simulink model "qiita3"  (R2019a)
settings: Solver=FixedStepDiscrete  StartTime=0.0  StopTime=Inf  FixedStep=0.001  RelTol=1e-3  EnableMultiTasking=on
libraries: robotlib x12, simulink x5
settings Model: Creator=tatsuyai  LastModifiedBy=tatsuyai
settings SolverCC: PositivePriorityOrder=on
settings OptimizationCC: EnhancedBackFolding=on  PassReuseOutputArgsAs=Individual arguments  ZeroExternalMemoryAtStartup=off  ZeroInternalMemoryAtStartup=off  MaxStackSize=64  OptimizeBlockOrder=speed  DifferentSizesBufferReuse=on  OptimizationCustomize=off
settings DebuggingCC: ParameterTunabilityLossMsg=error
settings HardwareCC: ProdBitPerLong=64  ProdBitPerPointer=32  ProdBitPerSizeT=32  ProdBitPerPtrDiffT=32  ProdLargestAtomicInteger=Long  ProdLargestAtomicFloat=Double  ProdWordSize=32  ProdHWDeviceType=ARM Compatible->ARM Cortex  TargetBitPerLong=64  UseEmbeddedCoderFeatures=off  UseSimulinkCoderFeatures=off
settings RTWCC: SystemTargetFile=ert.tlc  HardwareBoard=Raspberry Pi - Robot Operating System (ROS)  TLCOptions="-aInlineSetEventsForThisBaseRateFcn=TLC_FALSE -aSuppressMultiTaskScheduler=TLC_FALSE  -aRateBasedStepFcn=0"  TemplateMakefile=ert_default_tmf  GenerateReport=on  Toolchain=Catkin  BuildConfiguration=Faster Runs  IncludeHyperlinkInReport=on  LaunchReport=on  TargetLang=C++  GenerateTraceInfo=on  GenerateTraceReport=on  GenerateTraceReportSl=on  GenerateTraceReportSf=on  GenerateTraceReportEml=on
settings CodeAppCC: ForceParamTrailComments=on  IgnoreCustomStorageClasses=off  OperatorAnnotations=on  SimulinkDataObjDesc=on  SFDataObjDesc=on  InsertBlockDesc=on
settings ERTTargetCC: SupportNonInlinedSFcns=on  SupportVariableSizeSignals=on

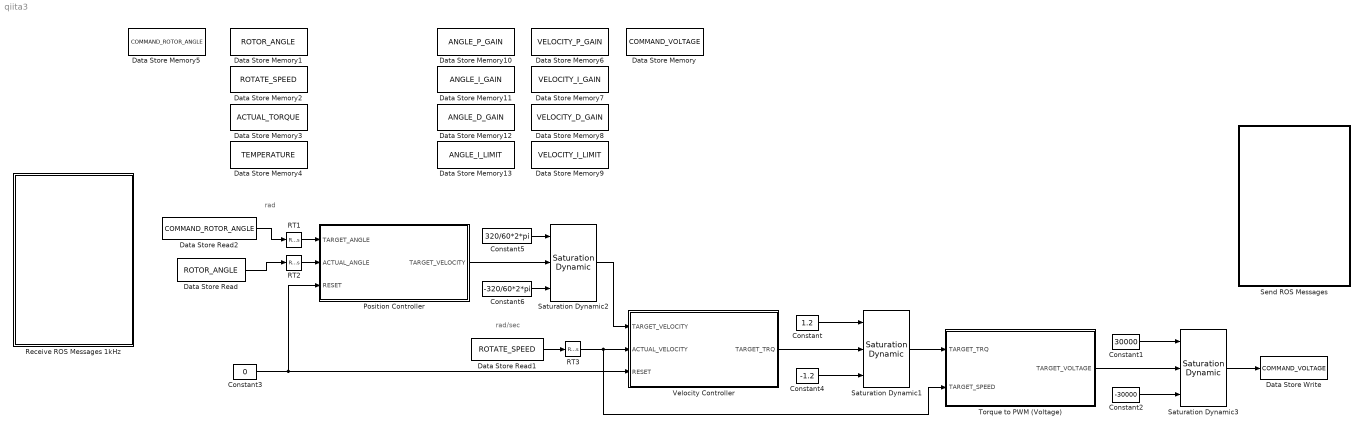
== system qiita3 ==
  note: rad
  note: rad/sec
  Constant : Constant  Value=1.2
  Constant1 : Constant  Value=30000
  Constant2 : Constant  Value=-30000
  Constant3 : Constant  Value=0
  Constant4 : Constant  Value=-1.2
  Constant5 : Constant  Value=320/60*2*pi
  Constant6 : Constant  Value=-320/60*2*pi
  Data Store Memory : DataStoreMemory  DataStoreName=COMMAND_VOLTAGE  ReadBeforeWriteMsg=warning  WriteAfterWriteMsg=warning  WriteAfterReadMsg=warning  ShowAdditionalParam=off
      settings: RTWStateStorageClass=ExportedGlobal
  Data Store Memory1 : DataStoreMemory  DataStoreName=ROTOR_ANGLE  ReadBeforeWriteMsg=warning  WriteAfterWriteMsg=warning  WriteAfterReadMsg=warning  ShowAdditionalParam=off
      settings: RTWStateStorageClass=ExportedGlobal
  Data Store Memory10 : DataStoreMemory  DataStoreName=ANGLE_P_GAIN  ReadBeforeWriteMsg=warning  WriteAfterWriteMsg=warning  WriteAfterReadMsg=warning  ShowAdditionalParam=off
      settings: RTWStateStorageClass=ExportedGlobal
  Data Store Memory11 : DataStoreMemory  DataStoreName=ANGLE_I_GAIN  ReadBeforeWriteMsg=warning  WriteAfterWriteMsg=warning  WriteAfterReadMsg=warning  ShowAdditionalParam=off
      settings: RTWStateStorageClass=ExportedGlobal
  Data Store Memory12 : DataStoreMemory  DataStoreName=ANGLE_D_GAIN  ReadBeforeWriteMsg=warning  WriteAfterWriteMsg=warning  WriteAfterReadMsg=warning  ShowAdditionalParam=off
      settings: RTWStateStorageClass=ExportedGlobal
  Data Store Memory13 : DataStoreMemory  DataStoreName=ANGLE_I_LIMIT  ReadBeforeWriteMsg=warning  WriteAfterWriteMsg=warning  WriteAfterReadMsg=warning  ShowAdditionalParam=off
      settings: RTWStateStorageClass=ExportedGlobal
  Data Store Memory2 : DataStoreMemory  DataStoreName=ROTATE_SPEED  ReadBeforeWriteMsg=warning  WriteAfterWriteMsg=warning  WriteAfterReadMsg=warning  ShowAdditionalParam=off
      settings: RTWStateStorageClass=ExportedGlobal
  Data Store Memory3 : DataStoreMemory  DataStoreName=ACTUAL_TORQUE  ReadBeforeWriteMsg=warning  WriteAfterWriteMsg=warning  WriteAfterReadMsg=warning  ShowAdditionalParam=off
      settings: RTWStateStorageClass=ExportedGlobal
  Data Store Memory4 : DataStoreMemory  DataStoreName=TEMPERATURE  ReadBeforeWriteMsg=warning  WriteAfterWriteMsg=warning  WriteAfterReadMsg=warning  ShowAdditionalParam=off
      settings: RTWStateStorageClass=ExportedGlobal
  Data Store Memory5 : DataStoreMemory  DataStoreName=COMMAND_ROTOR_ANGLE  ReadBeforeWriteMsg=warning  WriteAfterWriteMsg=warning  WriteAfterReadMsg=warning  ShowAdditionalParam=off
      settings: RTWStateStorageClass=ExportedGlobal
  Data Store Memory6 : DataStoreMemory  DataStoreName=VELOCITY_P_GAIN  ReadBeforeWriteMsg=warning  WriteAfterWriteMsg=warning  WriteAfterReadMsg=warning  ShowAdditionalParam=off
      settings: RTWStateStorageClass=ExportedGlobal
  Data Store Memory7 : DataStoreMemory  DataStoreName=VELOCITY_I_GAIN  ReadBeforeWriteMsg=warning  WriteAfterWriteMsg=warning  WriteAfterReadMsg=warning  ShowAdditionalParam=off
      settings: RTWStateStorageClass=ExportedGlobal
  Data Store Memory8 : DataStoreMemory  DataStoreName=VELOCITY_D_GAIN  ReadBeforeWriteMsg=warning  WriteAfterWriteMsg=warning  WriteAfterReadMsg=warning  ShowAdditionalParam=off
      settings: RTWStateStorageClass=ExportedGlobal
  Data Store Memory9 : DataStoreMemory  DataStoreName=VELOCITY_I_LIMIT  ReadBeforeWriteMsg=warning  WriteAfterWriteMsg=warning  WriteAfterReadMsg=warning  ShowAdditionalParam=off
      settings: RTWStateStorageClass=ExportedGlobal
  Data Store Read : DataStoreRead  DataStoreName=ROTOR_ANGLE
  Data Store Read1 : DataStoreRead  DataStoreName=ROTATE_SPEED
  Data Store Read2 : DataStoreRead  DataStoreName=COMMAND_ROTOR_ANGLE
  Data Store Write : DataStoreWrite  DataStoreName=COMMAND_VOLTAGE
  Position Controller : Subsystem  TreatAsAtomicUnit=on  SystemSampleTime=0.01
  RT1 : RateTransition  Deterministic=off  OutPortSampleTime=0.01
  RT2 : RateTransition  Deterministic=off  OutPortSampleTime=0.01
  RT3 : RateTransition  Deterministic=off  OutPortSampleTime=0.01
  Receive ROS Messages 1kHz : Subsystem  TreatAsAtomicUnit=on  SystemSampleTime=0.001
  Saturation Dynamic1 : simulink/Discontinuities/Saturation Dynamic  OutMin=[]  OutMax=[]  OutDataTypeStr=Inherit: Same as second input  OutDataType=fixdt(1, 16)  OutScaling=2^-10  DoSatur=off
  Saturation Dynamic2 : simulink/Discontinuities/Saturation Dynamic  OutMin=[]  OutMax=[]  OutDataTypeStr=Inherit: Same as second input  OutDataType=fixdt(1, 16)  OutScaling=2^-10  DoSatur=off
  Saturation Dynamic3 : simulink/Discontinuities/Saturation Dynamic  OutMin=[]  OutMax=[]  OutDataTypeStr=Inherit: Same as second input  OutDataType=fixdt(1, 16)  OutScaling=2^-10  DoSatur=off
  Send ROS Messages : Subsystem  TreatAsAtomicUnit=on  SystemSampleTime=0.01
  Torque to PWM (Voltage) : Subsystem  TreatAsAtomicUnit=on  SystemSampleTime=0.01
  Velocity Controller : Subsystem  TreatAsAtomicUnit=on  SystemSampleTime=0.01
  wires:
  Constant/1 -> Saturation Dynamic1/1
  Velocity Controller/1(TARGET_TRQ) -> Saturation Dynamic1/2
  Constant4/1 -> Saturation Dynamic1/3
  Saturation Dynamic1/1 -> Torque to PWM (Voltage)/1(TARGET_TRQ)
  Position Controller/1(TARGET_VELOCITY) -> Saturation Dynamic2/2
  Constant6/1 -> Saturation Dynamic2/3
  Constant5/1 -> Saturation Dynamic2/1
  Saturation Dynamic2/1 -> Velocity Controller/1(TARGET_VELOCITY)
  Data Store Read/1 -> RT2/1
  Data Store Read1/1 -> RT3/1
  Saturation Dynamic3/1 -> Data Store Write/1
  Torque to PWM (Voltage)/1(TARGET_VOLTAGE) -> Saturation Dynamic3/2
  Constant2/1 -> Saturation Dynamic3/3
  Constant1/1 -> Saturation Dynamic3/1
  Data Store Read2/1 -> RT1/1
  Constant3/1 -> Velocity Controller/3(RESET), Position Controller/3(RESET)
  RT1/1 -> Position Controller/1(TARGET_ANGLE)
  RT2/1 -> Position Controller/2(ACTUAL_ANGLE)
  RT3/1 -> Velocity Controller/2(ACTUAL_VELOCITY), Torque to PWM (Voltage)/2(TARGET_SPEED)

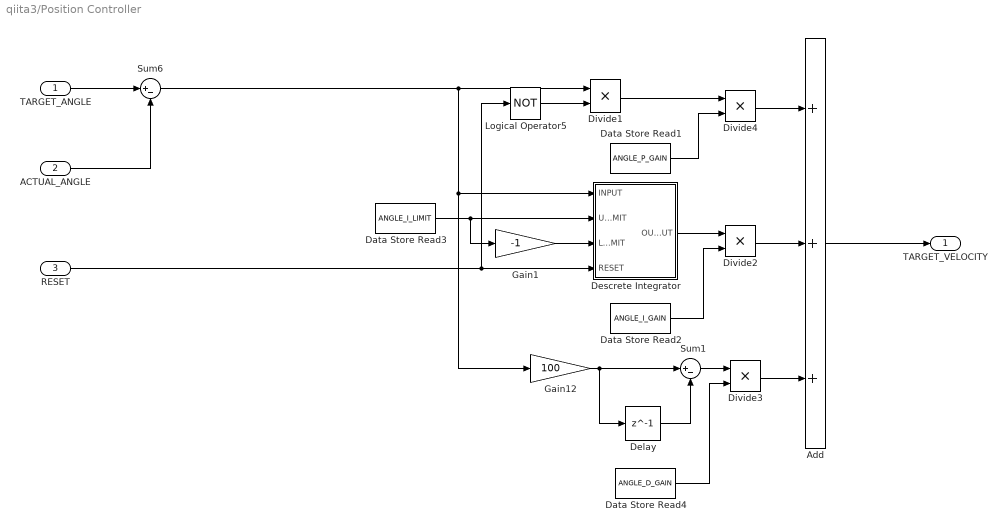
== system qiita3/Position Controller ==
  TARGET_ANGLE : Inport
  ACTUAL_ANGLE : Inport  Port=2
  RESET : Inport  Port=3
  Add : Sum  Inputs=+++
  Data Store Read1 : DataStoreRead  DataStoreName=ANGLE_P_GAIN
  Data Store Read2 : DataStoreRead  DataStoreName=ANGLE_I_GAIN
  Data Store Read3 : DataStoreRead  DataStoreName=ANGLE_I_LIMIT
  Data Store Read4 : DataStoreRead  DataStoreName=ANGLE_D_GAIN
  Delay : Delay  DelayLength=1
  Descrete Integrator : Subsystem  mask(DISCRETE INTEGRATOR){sampling_time=0.01}
      mask prompts: sampling_time "Sampling Time: (-1) is not valid"
      settings: CopyFcn=set_param(gcbh,'LinkStatus','none')
  Divide{1..4} (4 alike) : Product  Inputs=**
  Gain1 : Gain  Gain=-1
  Gain12 : Gain  Gain=100
  Logical Operator5 : Logic  Operator=NOT  AllPortsSameDT=off  OutDataTypeStr=boolean
  Sum1 : Sum  Inputs=|+-
  Sum6 : Sum  Inputs=|+-
  TARGET_VELOCITY : Outport
  wires:
  Gain1/1 -> Descrete Integrator/3(LOWER LIMIT)
  TARGET_ANGLE/1 -> Sum6/1
  Data Store Read2/1 -> Divide2/2
  Descrete Integrator/1(OUTPUT) -> Divide2/1
  Logical Operator5/1 -> Divide1/2
  Divide1/1 -> Divide4/1
  Data Store Read1/1 -> Divide4/2
  Data Store Read3/1 -> Gain1/1, Descrete Integrator/2(UPPER LIMIT)
  RESET/1 -> Logical Operator5/1, Descrete Integrator/4(RESET)
  ACTUAL_ANGLE/1 -> Sum6/2
  Divide2/1 -> Add/2
  Divide4/1 -> Add/1
  Delay/1 -> Sum1/2
  Sum6/1 -> Gain12/1, Descrete Integrator/1(INPUT), Divide1/1
  Gain12/1 -> Delay/1, Sum1/1
  Sum1/1 -> Divide3/1
  Add/1 -> TARGET_VELOCITY/1
  Divide3/1 -> Add/3
  Data Store Read4/1 -> Divide3/2

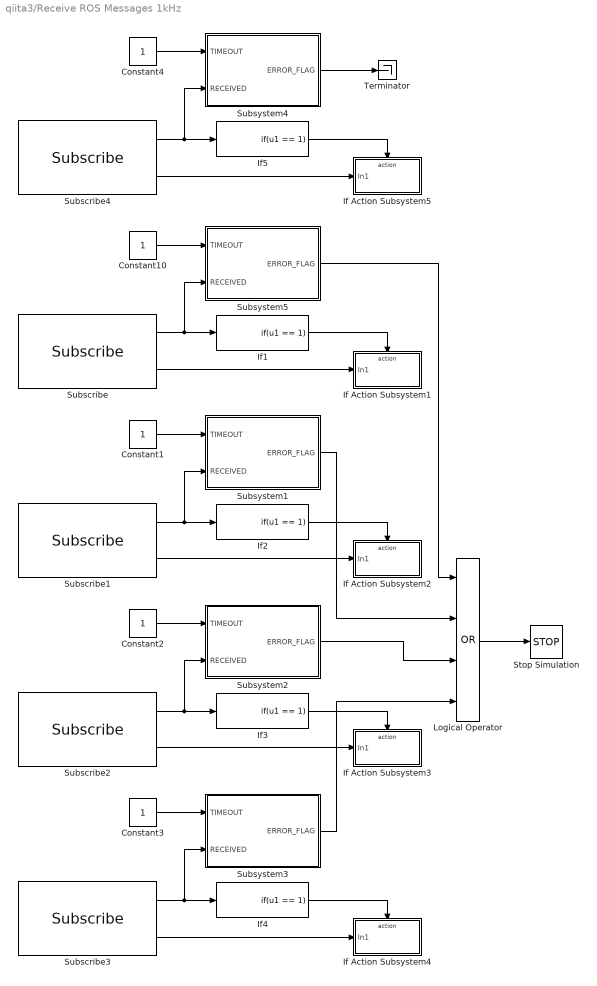
== system qiita3/Receive ROS Messages 1kHz ==
  Constant{1..4,10} (5 alike) : Constant
  If Action Subsystem1 : Subsystem  TreatAsAtomicUnit=on
  If Action Subsystem2 : Subsystem  TreatAsAtomicUnit=on
  If Action Subsystem3 : Subsystem  TreatAsAtomicUnit=on
  If Action Subsystem4 : Subsystem  TreatAsAtomicUnit=on
  If Action Subsystem5 : Subsystem  TreatAsAtomicUnit=on
  If{1..5} (5 alike) : If  IfExpression=u1 == 1  ShowElse=off
  Logical Operator : Logic  Operator=OR  Inputs=4  AllPortsSameDT=off  OutDataTypeStr=boolean
  Stop Simulation : Stop
  Subscribe : robotlib/Subscribe  topicSource=Specify your own  topic=/gm6020_1/rotor_angle  messageType=std_msgs/Float64  sampleTime=-1  messageQueueLength=1
      settings: SourceProductName=ROS Toolbox
  Subscribe1 : robotlib/Subscribe  topicSource=Specify your own  topic=/gm6020_1/rotate_speed  messageType=std_msgs/Float64  sampleTime=-1  messageQueueLength=1
      settings: SourceProductName=ROS Toolbox
  Subscribe2 : robotlib/Subscribe  topicSource=Specify your own  topic=/gm6020_1/actual_trq  messageType=std_msgs/Float64  sampleTime=-1  messageQueueLength=1
      settings: SourceProductName=ROS Toolbox
  Subscribe3 : robotlib/Subscribe  topicSource=Specify your own  topic=/gm6020_1/temp  messageType=std_msgs/Int8  sampleTime=-1  messageQueueLength=1
      settings: SourceProductName=ROS Toolbox
  Subscribe4 : robotlib/Subscribe  topicSource=Specify your own  topic=/gm6020_1/cmd_rotor_angle  messageType=std_msgs/Float64  sampleTime=-1  messageQueueLength=1
      settings: SourceProductName=ROS Toolbox
  Subsystem1 : Subsystem
  Subsystem2 : Subsystem
  Subsystem3 : Subsystem
  Subsystem4 : Subsystem
  Subsystem5 : Subsystem
  Terminator : Terminator
  wires:
  Subsystem1/1(ERROR_FLAG) -> Logical Operator/2
  Subscribe2/2 -> If Action Subsystem3/1(In1)
  If2/1 -> If Action Subsystem2/Action
  Subscribe/1 -> Subsystem5/2(RECEIVED), If1/1
  Constant1/1 -> Subsystem1/1(TIMEOUT)
  Constant2/1 -> Subsystem2/1(TIMEOUT)
  Subsystem3/1(ERROR_FLAG) -> Logical Operator/4
  Subscribe2/1 -> Subsystem2/2(RECEIVED), If3/1
  If1/1 -> If Action Subsystem1/Action
  Subsystem2/1(ERROR_FLAG) -> Logical Operator/3
  Logical Operator/1 -> Stop Simulation/1
  If3/1 -> If Action Subsystem3/Action
  Subscribe1/1 -> Subsystem1/2(RECEIVED), If2/1
  Subscribe3/2 -> If Action Subsystem4/1(In1)
  Constant3/1 -> Subsystem3/1(TIMEOUT)
  Subscribe/2 -> If Action Subsystem1/1(In1)
  If4/1 -> If Action Subsystem4/Action
  Subscribe1/2 -> If Action Subsystem2/1(In1)
  Subsystem5/1(ERROR_FLAG) -> Logical Operator/1
  Subscribe3/1 -> Subsystem3/2(RECEIVED), If4/1
  Constant10/1 -> Subsystem5/1(TIMEOUT)
  Subscribe4/1 -> Subsystem4/2(RECEIVED), If5/1
  If5/1 -> If Action Subsystem5/Action
  Subscribe4/2 -> If Action Subsystem5/1(In1)
  Constant4/1 -> Subsystem4/1(TIMEOUT)
  Subsystem4/1(ERROR_FLAG) -> Terminator/1

== system qiita3/Send ROS Messages ==
  Blank Message : robotlib/Blank Message  messageClass=Message  entityType=std_msgs/Int16  messageType=std_msgs/Int16  SampleTime=inf
      settings: SourceProductName=ROS Toolbox
  Bus Assignment : BusAssignment  AssignedSignals=Data
  Data Store Read2 : DataStoreRead  DataStoreName=COMMAND_VOLTAGE
  Data Type Conversion4 : DataTypeConversion  OutDataTypeStr=int16
  Publish : robotlib/Publish  topicSource=Specify your own  topic=/gm6020_1/cmd_voltage  messageType=std_msgs/Int16  messageQueueLength=1
      settings: SourceProductName=ROS Toolbox
  wires:
  Data Store Read2/1 -> Data Type Conversion4/1
  Bus Assignment/1 -> Publish/1
  Blank Message/1 -> Bus Assignment/1
  Data Type Conversion4/1 -> Bus Assignment/2

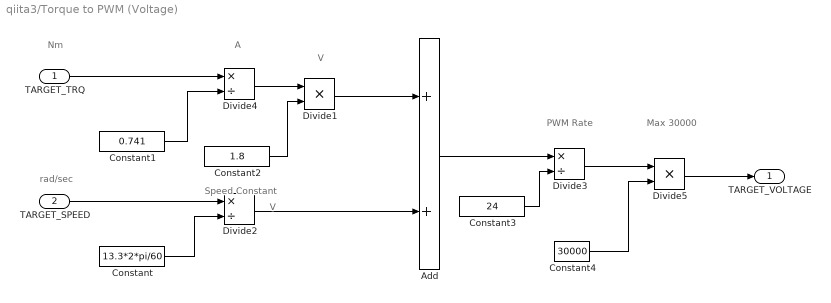
== system qiita3/Torque to PWM (Voltage) ==
  note: Nm
  note: A
  note: V
  note: PWM Rate
  note: Max 30000
  note: Speed Constant
  note: rad/sec
  note: V
  TARGET_TRQ : Inport
  TARGET_SPEED : Inport  Port=2
  Add : Sum
  Constant : Constant  Value=13.3*2*pi/60
  Constant1 : Constant  Value=0.741
  Constant2 : Constant  Value=1.8
  Constant3 : Constant  Value=24
  Constant4 : Constant  Value=30000
  Divide1 : Product  Inputs=**
  Divide2 : Product  Inputs=*/
  Divide3 : Product  Inputs=*/
  Divide4 : Product  Inputs=*/
  Divide5 : Product  Inputs=**
  TARGET_VOLTAGE : Outport
  wires:
  Constant1/1 -> Divide4/2
  TARGET_TRQ/1 -> Divide4/1
  TARGET_SPEED/1 -> Divide2/1
  Constant/1 -> Divide2/2
  Divide4/1 -> Divide1/1
  Divide2/1 -> Add/2
  Add/1 -> Divide3/1
  Divide1/1 -> Add/1
  Constant2/1 -> Divide1/2
  Divide3/1 -> Divide5/1
  Constant3/1 -> Divide3/2
  Divide5/1 -> TARGET_VOLTAGE/1
  Constant4/1 -> Divide5/2

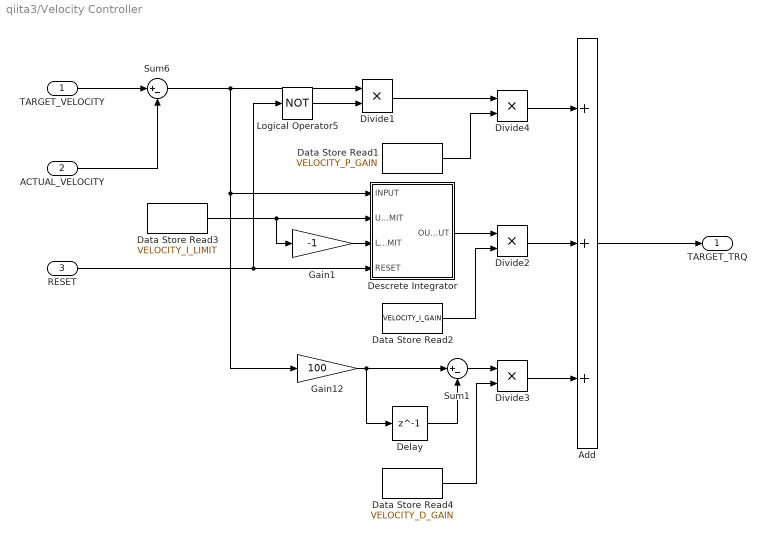
== system qiita3/Velocity Controller ==
  TARGET_VELOCITY : Inport
  ACTUAL_VELOCITY : Inport  Port=2
  RESET : Inport  Port=3
  Add : Sum  Inputs=+++
  Data Store Read1 : DataStoreRead  DataStoreName=VELOCITY_P_GAIN
  Data Store Read2 : DataStoreRead  DataStoreName=VELOCITY_I_GAIN
  Data Store Read3 : DataStoreRead  DataStoreName=VELOCITY_I_LIMIT
  Data Store Read4 : DataStoreRead  DataStoreName=VELOCITY_D_GAIN
  Delay : Delay  DelayLength=1
  Descrete Integrator : Subsystem  mask(DISCRETE INTEGRATOR){sampling_time=0.01}
      mask prompts: sampling_time "Sampling Time: (-1) is not valid"
      settings: CopyFcn=set_param(gcbh,'LinkStatus','none')
  Divide{1..4} (4 alike) : Product  Inputs=**
  Gain1 : Gain  Gain=-1
  Gain12 : Gain  Gain=100
  Logical Operator5 : Logic  Operator=NOT  AllPortsSameDT=off  OutDataTypeStr=boolean
  Sum1 : Sum  Inputs=|+-
  Sum6 : Sum  Inputs=|+-
  TARGET_TRQ : Outport
  wires:
  Sum1/1 -> Divide3/1
  Gain12/1 -> Sum1/1, Delay/1
  Sum6/1 -> Divide1/1, Descrete Integrator/1(INPUT), Gain12/1
  Delay/1 -> Sum1/2
  Divide4/1 -> Add/1
  Divide2/1 -> Add/2
  ACTUAL_VELOCITY/1 -> Sum6/2
  RESET/1 -> Descrete Integrator/4(RESET), Logical Operator5/1
  Data Store Read3/1 -> Descrete Integrator/2(UPPER LIMIT), Gain1/1
  Data Store Read1/1 -> Divide4/2
  Divide1/1 -> Divide4/1
  Logical Operator5/1 -> Divide1/2
  Descrete Integrator/1(OUTPUT) -> Divide2/1
  Data Store Read2/1 -> Divide2/2
  TARGET_VELOCITY/1 -> Sum6/1
  Gain1/1 -> Descrete Integrator/3(LOWER LIMIT)
  Divide3/1 -> Add/3
  Data Store Read4/1 -> Divide3/2
  Add/1 -> TARGET_TRQ/1

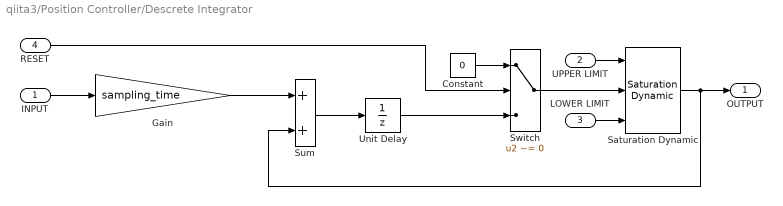
== system qiita3/Position Controller/Descrete Integrator ==
  INPUT : Inport
  UPPER LIMIT : Inport  Port=2
  LOWER LIMIT : Inport  Port=3
  RESET : Inport  Port=4
  Constant : Constant  Value=0
  Gain : Gain  Gain=sampling_time
  Saturation Dynamic : simulink/Discontinuities/Saturation Dynamic  OutMin=[]  OutMax=[]  OutDataTypeStr=Inherit: Same as second input  OutDataType=fixdt(1, 16)  OutScaling=2^-10  DoSatur=off
  Sum : Sum
  Switch : Switch  Criteria=u2 ~= 0
  Unit Delay : UnitDelay  SampleTime=-1  HasFrameUpgradeWarning=on
  OUTPUT : Outport
  wires:
  LOWER LIMIT/1 -> Saturation Dynamic/3
  UPPER LIMIT/1 -> Saturation Dynamic/1
  Constant/1 -> Switch/1
  RESET/1 -> Switch/2
  Switch/1 -> Saturation Dynamic/2
  Unit Delay/1 -> Switch/3
  INPUT/1 -> Gain/1
  Gain/1 -> Sum/1
  Sum/1 -> Unit Delay/1
  Saturation Dynamic/1 -> Sum/2, OUTPUT/1

== system qiita3/Receive ROS Messages 1kHz/If Action Subsystem1 ==
  In1 : Inport
  Action Port : ActionPort  ActionPortLabel=if(u1 == 1)
  Bus Selector : BusSelector  OutputSignals=Data
  Data Store Write : DataStoreWrite  DataStoreName=ROTOR_ANGLE
  wires:
  In1/1 -> Bus Selector/1
  Bus Selector/1 -> Data Store Write/1  "<Data>"

== system qiita3/Receive ROS Messages 1kHz/If Action Subsystem2 ==
  In1 : Inport
  Action Port : ActionPort  ActionPortLabel=if(u1 == 1)
  Bus Selector : BusSelector  OutputSignals=Data
  Data Store Write : DataStoreWrite  DataStoreName=ROTATE_SPEED
  wires:
  In1/1 -> Bus Selector/1
  Bus Selector/1 -> Data Store Write/1  "<Data>"

== system qiita3/Receive ROS Messages 1kHz/If Action Subsystem3 ==
  In1 : Inport
  Action Port : ActionPort  ActionPortLabel=if(u1 == 1)
  Bus Selector : BusSelector  OutputSignals=Data
  Data Store Write : DataStoreWrite  DataStoreName=ACTUAL_TORQUE
  wires:
  In1/1 -> Bus Selector/1
  Bus Selector/1 -> Data Store Write/1  "<Data>"

== system qiita3/Receive ROS Messages 1kHz/If Action Subsystem4 ==
  In1 : Inport
  Action Port : ActionPort  ActionPortLabel=if(u1 == 1)
  Bus Selector : BusSelector  OutputSignals=Data
  Data Store Write : DataStoreWrite  DataStoreName=TEMPERATURE
  wires:
  In1/1 -> Bus Selector/1
  Bus Selector/1 -> Data Store Write/1  "<Data>"

== system qiita3/Receive ROS Messages 1kHz/If Action Subsystem5 ==
  In1 : Inport
  Action Port : ActionPort  ActionPortLabel=if(u1 == 1)
  Bus Selector : BusSelector  OutputSignals=Data
  Data Store Write : DataStoreWrite  DataStoreName=COMMAND_ROTOR_ANGLE
  wires:
  In1/1 -> Bus Selector/1
  Bus Selector/1 -> Data Store Write/1  "<Data>"

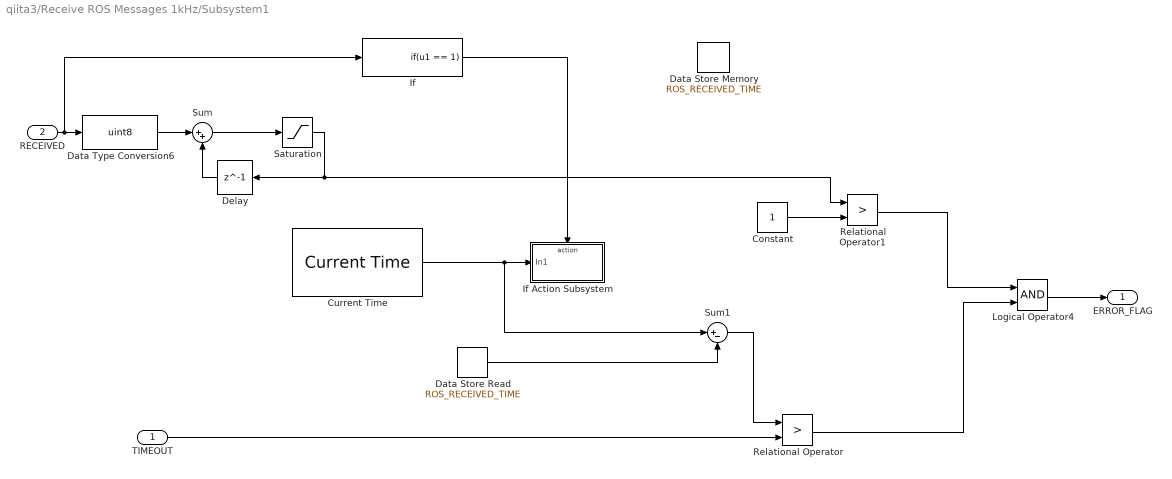
== system qiita3/Receive ROS Messages 1kHz/Subsystem1 ==
  TIMEOUT : Inport
  RECEIVED : Inport  Port=2
  Constant : Constant
  Current Time : robotlib/Current Time  OutputFormat=double  SampleTime=-1  ModelName=gm6020_pid_control_2019a
      settings: SourceProductName=Robotics System Toolbox  SourceProductBaseCode=RO
  Data Store Memory : DataStoreMemory  DataStoreName=ROS_RECEIVED_TIME  ReadBeforeWriteMsg=warning  WriteAfterWriteMsg=warning  WriteAfterReadMsg=warning  InitialValue=10  ShowAdditionalParam=off
  Data Store Read : DataStoreRead  DataStoreName=ROS_RECEIVED_TIME
  Data Type Conversion6 : DataTypeConversion  OutDataTypeStr=uint8
  Delay : Delay  DelayLength=1
  If : If  IfExpression=u1 == 1  ShowElse=off
  If Action Subsystem : Subsystem  TreatAsAtomicUnit=on
  Logical Operator4 : Logic  AllPortsSameDT=off  OutDataTypeStr=boolean
  Relational Operator : RelationalOperator  Operator=>  OutDataTypeStr=boolean  RndMeth=Simplest
  Relational Operator1 : RelationalOperator  Operator=>  OutDataTypeStr=boolean  RndMeth=Simplest
  Saturation : Saturate  UpperLimit=2  LowerLimit=0
  Sum : Sum  Inputs=|++
  Sum1 : Sum  Inputs=|+-
  ERROR_FLAG : Outport
  wires:
  Data Store Read/1 -> Sum1/2
  Sum1/1 -> Relational Operator/1
  RECEIVED/1 -> If/1, Data Type Conversion6/1
  Current Time/1 -> Sum1/1, If Action Subsystem/1(In1)
  If/1 -> If Action Subsystem/Action
  TIMEOUT/1 -> Relational Operator/2
  Relational Operator/1 -> Logical Operator4/2
  Saturation/1 -> Delay/1, Relational Operator1/1
  Sum/1 -> Saturation/1
  Delay/1 -> Sum/2
  Constant/1 -> Relational Operator1/2
  Logical Operator4/1 -> ERROR_FLAG/1
  Relational Operator1/1 -> Logical Operator4/1
  Data Type Conversion6/1 -> Sum/1

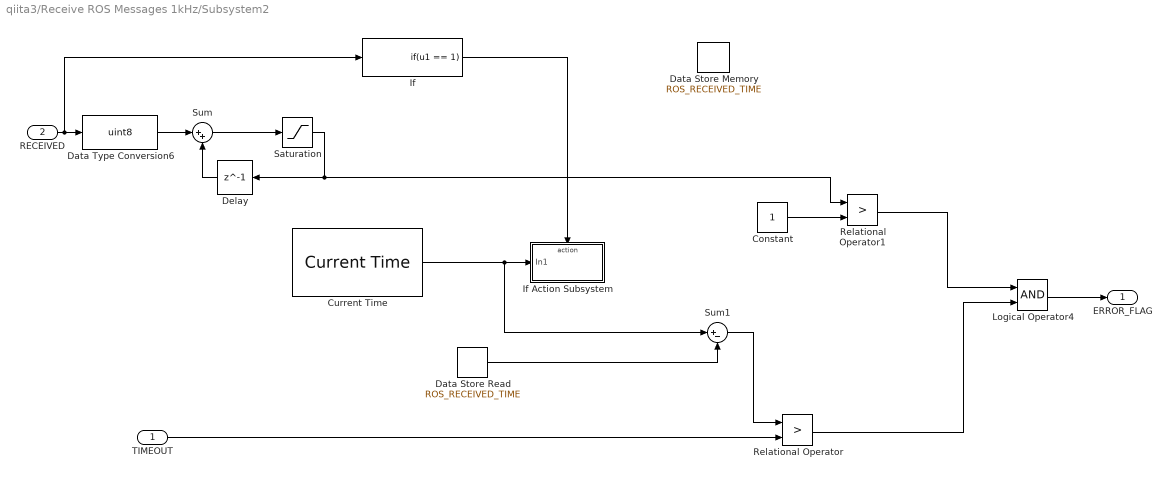
== system qiita3/Receive ROS Messages 1kHz/Subsystem2 ==
  TIMEOUT : Inport
  RECEIVED : Inport  Port=2
  Constant : Constant
  Current Time : robotlib/Current Time  OutputFormat=double  SampleTime=-1  ModelName=gm6020_pid_control_2019a
      settings: SourceProductName=Robotics System Toolbox  SourceProductBaseCode=RO
  Data Store Memory : DataStoreMemory  DataStoreName=ROS_RECEIVED_TIME  ReadBeforeWriteMsg=warning  WriteAfterWriteMsg=warning  WriteAfterReadMsg=warning  InitialValue=10  ShowAdditionalParam=off
  Data Store Read : DataStoreRead  DataStoreName=ROS_RECEIVED_TIME
  Data Type Conversion6 : DataTypeConversion  OutDataTypeStr=uint8
  Delay : Delay  DelayLength=1
  If : If  IfExpression=u1 == 1  ShowElse=off
  If Action Subsystem : Subsystem  TreatAsAtomicUnit=on
  Logical Operator4 : Logic  AllPortsSameDT=off  OutDataTypeStr=boolean
  Relational Operator : RelationalOperator  Operator=>  OutDataTypeStr=boolean  RndMeth=Simplest
  Relational Operator1 : RelationalOperator  Operator=>  OutDataTypeStr=boolean  RndMeth=Simplest
  Saturation : Saturate  UpperLimit=2  LowerLimit=0
  Sum : Sum  Inputs=|++
  Sum1 : Sum  Inputs=|+-
  ERROR_FLAG : Outport
  wires:
  Data Store Read/1 -> Sum1/2
  Sum1/1 -> Relational Operator/1
  RECEIVED/1 -> If/1, Data Type Conversion6/1
  Current Time/1 -> Sum1/1, If Action Subsystem/1(In1)
  If/1 -> If Action Subsystem/Action
  TIMEOUT/1 -> Relational Operator/2
  Relational Operator/1 -> Logical Operator4/2
  Saturation/1 -> Delay/1, Relational Operator1/1
  Sum/1 -> Saturation/1
  Delay/1 -> Sum/2
  Constant/1 -> Relational Operator1/2
  Logical Operator4/1 -> ERROR_FLAG/1
  Relational Operator1/1 -> Logical Operator4/1
  Data Type Conversion6/1 -> Sum/1

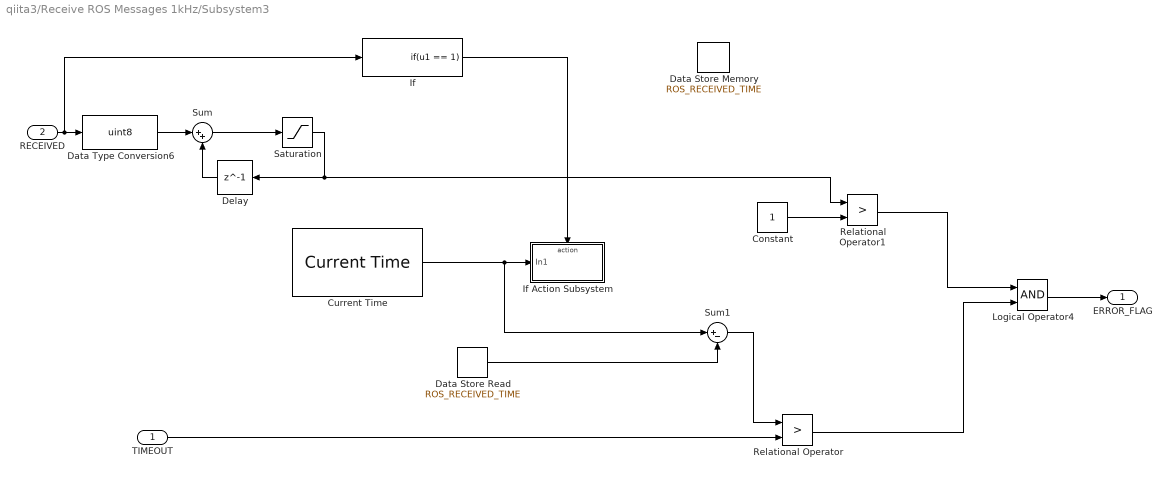
== system qiita3/Receive ROS Messages 1kHz/Subsystem3 ==
  TIMEOUT : Inport
  RECEIVED : Inport  Port=2
  Constant : Constant
  Current Time : robotlib/Current Time  OutputFormat=double  SampleTime=-1  ModelName=gm6020_pid_control_2019a
      settings: SourceProductName=Robotics System Toolbox  SourceProductBaseCode=RO
  Data Store Memory : DataStoreMemory  DataStoreName=ROS_RECEIVED_TIME  ReadBeforeWriteMsg=warning  WriteAfterWriteMsg=warning  WriteAfterReadMsg=warning  InitialValue=10  ShowAdditionalParam=off
  Data Store Read : DataStoreRead  DataStoreName=ROS_RECEIVED_TIME
  Data Type Conversion6 : DataTypeConversion  OutDataTypeStr=uint8
  Delay : Delay  DelayLength=1
  If : If  IfExpression=u1 == 1  ShowElse=off
  If Action Subsystem : Subsystem  TreatAsAtomicUnit=on
  Logical Operator4 : Logic  AllPortsSameDT=off  OutDataTypeStr=boolean
  Relational Operator : RelationalOperator  Operator=>  OutDataTypeStr=boolean  RndMeth=Simplest
  Relational Operator1 : RelationalOperator  Operator=>  OutDataTypeStr=boolean  RndMeth=Simplest
  Saturation : Saturate  UpperLimit=2  LowerLimit=0
  Sum : Sum  Inputs=|++
  Sum1 : Sum  Inputs=|+-
  ERROR_FLAG : Outport
  wires:
  Data Store Read/1 -> Sum1/2
  Sum1/1 -> Relational Operator/1
  RECEIVED/1 -> If/1, Data Type Conversion6/1
  Current Time/1 -> Sum1/1, If Action Subsystem/1(In1)
  If/1 -> If Action Subsystem/Action
  TIMEOUT/1 -> Relational Operator/2
  Relational Operator/1 -> Logical Operator4/2
  Saturation/1 -> Delay/1, Relational Operator1/1
  Sum/1 -> Saturation/1
  Delay/1 -> Sum/2
  Constant/1 -> Relational Operator1/2
  Logical Operator4/1 -> ERROR_FLAG/1
  Relational Operator1/1 -> Logical Operator4/1
  Data Type Conversion6/1 -> Sum/1

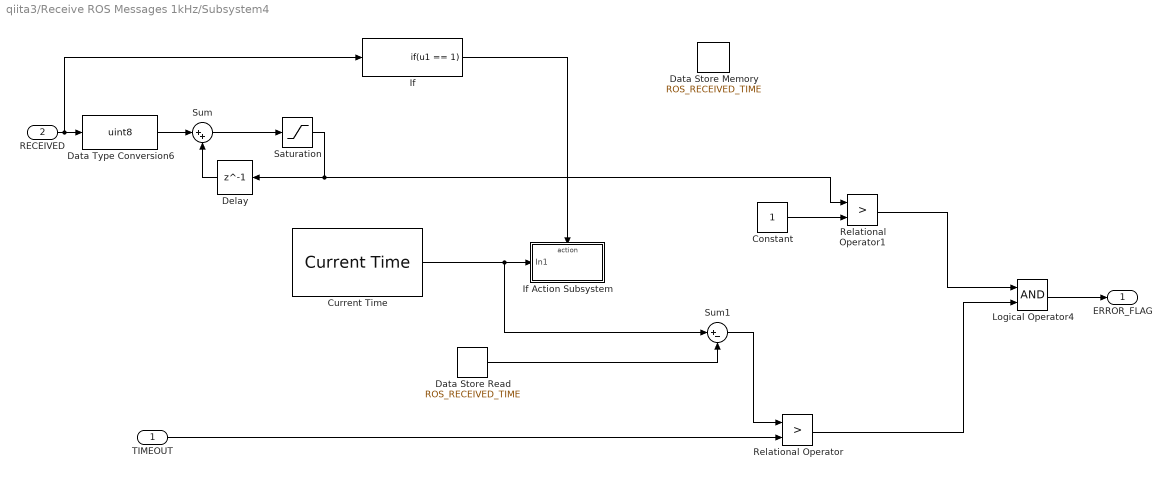
== system qiita3/Receive ROS Messages 1kHz/Subsystem4 ==
  TIMEOUT : Inport
  RECEIVED : Inport  Port=2
  Constant : Constant
  Current Time : robotlib/Current Time  OutputFormat=double  SampleTime=-1  ModelName=gm6020_pid_control_2019a
      settings: SourceProductName=Robotics System Toolbox  SourceProductBaseCode=RO
  Data Store Memory : DataStoreMemory  DataStoreName=ROS_RECEIVED_TIME  ReadBeforeWriteMsg=warning  WriteAfterWriteMsg=warning  WriteAfterReadMsg=warning  InitialValue=10  ShowAdditionalParam=off
  Data Store Read : DataStoreRead  DataStoreName=ROS_RECEIVED_TIME
  Data Type Conversion6 : DataTypeConversion  OutDataTypeStr=uint8
  Delay : Delay  DelayLength=1
  If : If  IfExpression=u1 == 1  ShowElse=off
  If Action Subsystem : Subsystem  TreatAsAtomicUnit=on
  Logical Operator4 : Logic  AllPortsSameDT=off  OutDataTypeStr=boolean
  Relational Operator : RelationalOperator  Operator=>  OutDataTypeStr=boolean  RndMeth=Simplest
  Relational Operator1 : RelationalOperator  Operator=>  OutDataTypeStr=boolean  RndMeth=Simplest
  Saturation : Saturate  UpperLimit=2  LowerLimit=0
  Sum : Sum  Inputs=|++
  Sum1 : Sum  Inputs=|+-
  ERROR_FLAG : Outport
  wires:
  Data Store Read/1 -> Sum1/2
  Sum1/1 -> Relational Operator/1
  RECEIVED/1 -> If/1, Data Type Conversion6/1
  Current Time/1 -> Sum1/1, If Action Subsystem/1(In1)
  If/1 -> If Action Subsystem/Action
  TIMEOUT/1 -> Relational Operator/2
  Relational Operator/1 -> Logical Operator4/2
  Saturation/1 -> Delay/1, Relational Operator1/1
  Sum/1 -> Saturation/1
  Delay/1 -> Sum/2
  Constant/1 -> Relational Operator1/2
  Logical Operator4/1 -> ERROR_FLAG/1
  Relational Operator1/1 -> Logical Operator4/1
  Data Type Conversion6/1 -> Sum/1

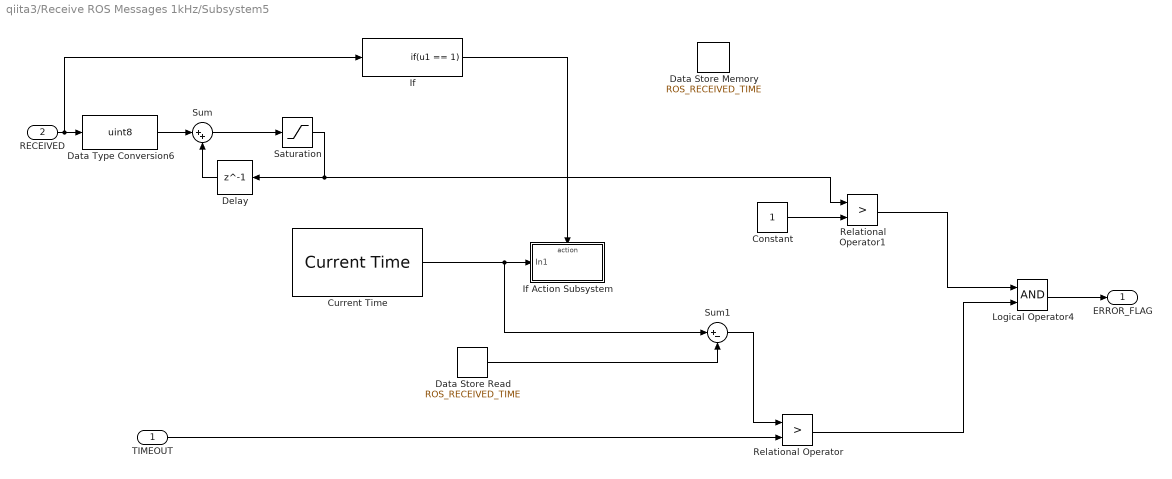
== system qiita3/Receive ROS Messages 1kHz/Subsystem5 ==
  TIMEOUT : Inport
  RECEIVED : Inport  Port=2
  Constant : Constant
  Current Time : robotlib/Current Time  OutputFormat=double  SampleTime=-1  ModelName=gm6020_pid_control_2019a
      settings: SourceProductName=Robotics System Toolbox  SourceProductBaseCode=RO
  Data Store Memory : DataStoreMemory  DataStoreName=ROS_RECEIVED_TIME  ReadBeforeWriteMsg=warning  WriteAfterWriteMsg=warning  WriteAfterReadMsg=warning  InitialValue=10  ShowAdditionalParam=off
  Data Store Read : DataStoreRead  DataStoreName=ROS_RECEIVED_TIME
  Data Type Conversion6 : DataTypeConversion  OutDataTypeStr=uint8
  Delay : Delay  DelayLength=1
  If : If  IfExpression=u1 == 1  ShowElse=off
  If Action Subsystem : Subsystem  TreatAsAtomicUnit=on
  Logical Operator4 : Logic  AllPortsSameDT=off  OutDataTypeStr=boolean
  Relational Operator : RelationalOperator  Operator=>  OutDataTypeStr=boolean  RndMeth=Simplest
  Relational Operator1 : RelationalOperator  Operator=>  OutDataTypeStr=boolean  RndMeth=Simplest
  Saturation : Saturate  UpperLimit=2  LowerLimit=0
  Sum : Sum  Inputs=|++
  Sum1 : Sum  Inputs=|+-
  ERROR_FLAG : Outport
  wires:
  Data Store Read/1 -> Sum1/2
  Sum1/1 -> Relational Operator/1
  RECEIVED/1 -> If/1, Data Type Conversion6/1
  Current Time/1 -> Sum1/1, If Action Subsystem/1(In1)
  If/1 -> If Action Subsystem/Action
  TIMEOUT/1 -> Relational Operator/2
  Relational Operator/1 -> Logical Operator4/2
  Saturation/1 -> Delay/1, Relational Operator1/1
  Sum/1 -> Saturation/1
  Delay/1 -> Sum/2
  Constant/1 -> Relational Operator1/2
  Logical Operator4/1 -> ERROR_FLAG/1
  Relational Operator1/1 -> Logical Operator4/1
  Data Type Conversion6/1 -> Sum/1

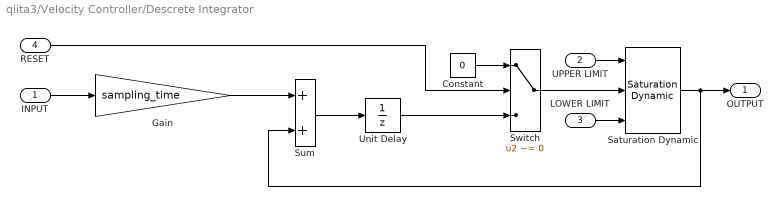
== system qiita3/Velocity Controller/Descrete Integrator ==
  INPUT : Inport
  UPPER LIMIT : Inport  Port=2
  LOWER LIMIT : Inport  Port=3
  RESET : Inport  Port=4
  Constant : Constant  Value=0
  Gain : Gain  Gain=sampling_time
  Saturation Dynamic : simulink/Discontinuities/Saturation Dynamic  OutMin=[]  OutMax=[]  OutDataTypeStr=Inherit: Same as second input  OutDataType=fixdt(1, 16)  OutScaling=2^-10  DoSatur=off
  Sum : Sum
  Switch : Switch  Criteria=u2 ~= 0
  Unit Delay : UnitDelay  SampleTime=-1  HasFrameUpgradeWarning=on
  OUTPUT : Outport
  wires:
  LOWER LIMIT/1 -> Saturation Dynamic/3
  UPPER LIMIT/1 -> Saturation Dynamic/1
  Constant/1 -> Switch/1
  RESET/1 -> Switch/2
  Switch/1 -> Saturation Dynamic/2
  Unit Delay/1 -> Switch/3
  INPUT/1 -> Gain/1
  Gain/1 -> Sum/1
  Sum/1 -> Unit Delay/1
  Saturation Dynamic/1 -> Sum/2, OUTPUT/1

== system qiita3/Receive ROS Messages 1kHz/Subsystem1/If Action Subsystem ==
  In1 : Inport
  Action Port : ActionPort  ActionPortLabel=if(u1 == 1)
  Data Store Write : DataStoreWrite  DataStoreName=ROS_RECEIVED_TIME
  wires:
  In1/1 -> Data Store Write/1

== system qiita3/Receive ROS Messages 1kHz/Subsystem2/If Action Subsystem ==
  In1 : Inport
  Action Port : ActionPort  ActionPortLabel=if(u1 == 1)
  Data Store Write : DataStoreWrite  DataStoreName=ROS_RECEIVED_TIME
  wires:
  In1/1 -> Data Store Write/1

== system qiita3/Receive ROS Messages 1kHz/Subsystem3/If Action Subsystem ==
  In1 : Inport
  Action Port : ActionPort  ActionPortLabel=if(u1 == 1)
  Data Store Write : DataStoreWrite  DataStoreName=ROS_RECEIVED_TIME
  wires:
  In1/1 -> Data Store Write/1

== system qiita3/Receive ROS Messages 1kHz/Subsystem4/If Action Subsystem ==
  In1 : Inport
  Action Port : ActionPort  ActionPortLabel=if(u1 == 1)
  Data Store Write : DataStoreWrite  DataStoreName=ROS_RECEIVED_TIME
  wires:
  In1/1 -> Data Store Write/1

== system qiita3/Receive ROS Messages 1kHz/Subsystem5/If Action Subsystem ==
  In1 : Inport
  Action Port : ActionPort  ActionPortLabel=if(u1 == 1)
  Data Store Write : DataStoreWrite  DataStoreName=ROS_RECEIVED_TIME
  wires:
  In1/1 -> Data Store Write/1
